simulink model "houle_model"  (R2025b)
settings: Solver=VariableStepAuto  StartTime=0.0  StopTime=30  RelTol=1e-3
values from neighbouring files (symbols this model uses):
  g = 9.81    [RAO.m]    (also in variables.m)
  Krao = 0.3    [RAO.m]    (also in variables.m = 100)
  Kw = 2*lambda*w0*sigma    [PM_spectrum.m]    (also in RAO.m; variables.m)
  lambda = 0.26    [PM_spectrum.m]    (also in RAO.m; variables.m)
  rho = 1025    [RAO.m]    (also in variables.m)
  w0 = 1.4    [PM_spectrum.m]    (also in RAO.m; variables.m)
  wR = 0.8    [RAO.m]    (also in variables.m)
  zeta = 0.25    [RAO.m]    (also in variables.m)
libraries: simulink x1
settings Model: Creator=hmbon  LastModifiedBy=flo

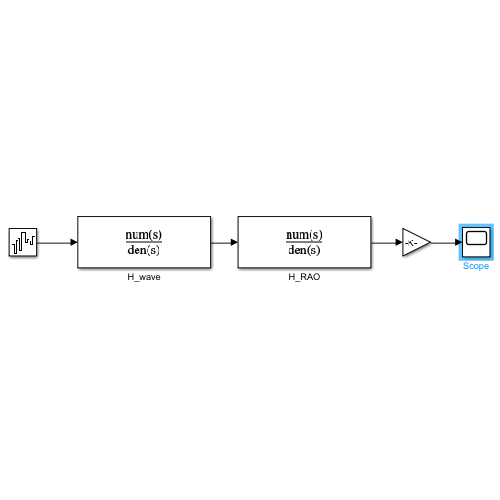
[thumbnail: Simulink's stored preview of the top-level diagram]
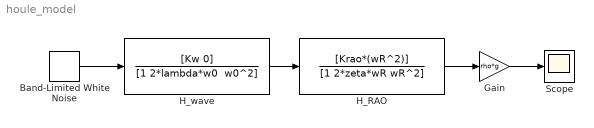
== system houle_model ==
  Band-Limited White Noise : simulink/Sources/Band-Limited White Noise  Cov=[0.1]  Ts=0.1  seed=[23341]
  Gain : Gain  Gain=rho*g
  H_RAO : TransferFcn  Numerator=[Krao*(wR^2)]  Denominator=[1 2*zeta*wR wR^2]
  H_wave : TransferFcn  Numerator=[Kw 0]  Denominator="[1 2*lambda*w0  w0^2]"
  Scope : Scope
      settings: ActiveDisplayYMinimum=-463.40253070202738  ActiveDisplayYMaximum=491.70262321441817
  wires:
  Band-Limited White Noise/1 -> H_wave/1
  H_wave/1 -> H_RAO/1
  H_RAO/1 -> Gain/1
  Gain/1 -> Scope/1
